simulink model "SimParking"  (R2017b)
settings: Solver=VariableStepAuto  StartTime=0.0  StopTime=1761  RelTol=1e-3
libraries: neural x1111
(part 21 of 60)

== system SimParking/10D- 100 100 100N/Layer 4/Delays 1 ==
  "p{4}" : Inport  PortDimensions=100  SampleTime=1
      mask Display: e = 0.06;c1 = [120 230 180]/255;c2 = ([120 230 180]+0)/(256+128);c3 = ([120 230 180]+128)/(256+128);patch([0 1 1 0],[0 0 1 1],c1);patch([0 1 1 1-e 1-e 0+e],[0 0 1 1-e 0+e 0+e],c2);patch([0 0 1 1-e 0+e 0+e],[0 1 1 1-e 1-e 0+e],c3);plot([0 1 1 0 0],[0 0 1 1 0]);
  mux : Mux  Inputs=1
      mask Display: e = 0.06;c1 = [120 150 230]/255;c2 = ([120 150 230]+0)/383;c3 = ([120 150 230]+128)/383;patch([0 1 1 0],[0 0 1 1],c1);patch([0 1 1 1-e 1-e 0+e],[0 0 1 1-e 0+e 0+e],c2);patch([0 0 1 1-e 0+e 0+e],[0 1 1 1-e 1-e 0+e],c3);plot([0 1 1 0 0],[0 0 1 1 0]);disp('Mux')
  "pd{4,3}" : Outport
      mask Display: e = 0.06;c1 = [120 230 180]/255;c2 = ([120 230 180]+0)/(256+128);c3 = ([120 230 180]+128)/(256+128);patch([0 1 1 0],[0 0 1 1],c1);patch([0 1 1 1-e 1-e 0+e],[0 0 1 1-e 0+e 0+e],c2);patch([0 0 1 1-e 0+e 0+e],[0 1 1 1-e 1-e 0+e],c3);plot([0 1 1 0 0],[0 0 1 1 0]);
  wires:
  "p{4}"/1 -> mux/1
  mux/1 -> "pd{4,3}"/1

== system SimParking/10D- 100 100 100N/Layer 4/LW{4,3} ==
  "ad{4,3}" : Inport  PortDimensions=100  SampleTime=1
      mask Display: e = 0.06;c1 = [120 230 180]/255;c2 = ([120 230 180]+0)/(256+128);c3 = ([120 230 180]+128)/(256+128);patch([0 1 1 0],[0 0 1 1],c1);patch([0 1 1 1-e 1-e 0+e],[0 0 1 1-e 0+e 0+e],c2);patch([0 0 1 1-e 0+e 0+e],[0 1 1 1-e 1-e 0+e],c3);plot([0 1 1 0 0],[0 0 1 1 0]);
  "IW{4,3}(1,:)'" : Constant  Value=[0.58065140864907160977992361949873156845569610595703125;-0.066112039002752365224324648806941695511341094970703125;1.0084944993814843883228604681789875030517578125;-0.9161011616738401475146247321390546858310699462890625;-0.61197886000859436084198250682675279676914215087890625;-0.96188175595466962608526273470488376915454864501953125;0.6658154478615332383384384229429997503757476806640625;0.253669306894615143033178128462168388068675994873046875;-0.047789102755492814111892840855944086797535419464111328125;0.2056930017197624582792059300118125975131988525390625;-0.788235313398349735081183098373003304004669189453125;0.81252383451202359054832413676194846630096435546875;0.880586120094551727532916629570536315441131591796875;0.310728251872029070934644323642714880406856536865234375;0.426423332746791949876552507703308947384357452392578125;-1.4378442695998241429578001771005801856517791748046875;-0.76862400698527266751369779740343801677227020263671875;-0.5367401396643509681183559223427437245845794677734375;0.1788804783596382730337381872232072055339813232421875;-0.483053438421408909420051713823340833187103271484375;0.260417950971423117767500343688880093395709991455078125;-0.63418149291668168832103447130066342651844024658203125;0.53082001579595605722516893365536816418170928955078125;0.6240704216430226214384902050369419157505035400390625;0.145969303182752307979086481282138265669345855712890625;-0.1372459925863576402083054972536046989262104034423828125;0.261788318191629232334349808297702111303806304931640625;-0.89483402758944607935376325258403085172176361083984375;0.400085557985017048476805712198256514966487884521484375;0.78620712071239751139728468842804431915283203125;-0.01616661136487627936642041959203197620809078216552734375;-0.319133591287700968397444967195042409002780914306640625;-0.5250450261200148016627053948468528687953948974609375;0.386346704245253913523328037626924924552440643310546875;-0.92227839555002699700736457089078612625598907470703125;-0.0933928000992329809815117869220557622611522674560546875;-0.0898344505816178473533994974786764942109584808349609375;0.03627984099991209132607394849401316605508327484130859375;0.213824804859598371908901981441886164247989654541015625;-0.71081554005856018019215980530134402215480804443359375;0.3213190743531277870914664163137786090373992919921875;-0.1329464050680488895750386291183531284332275390625;-0.7387626856994302659842333014239557087421417236328125;0.37941002852106742171400810548220761120319366455078125;-0.2280569383445431308476969434195780195295810699462890625;0.1898286392244080966751340611153864301741123199462890625;0.055918531953780638288353799225660623051226139068603515625;0.12618149731463901286332429663161747157573699951171875;-0.469304733579828992073856852584867738187313079833984375;0.45331359415498884146700220298953354358673095703125;-0.11241114545576184891029214441005024127662181854248046875;0.77149568550057912030837314887321554124355316162109375;0.5441020308254442827688990291790105402469635009765625;-0.4640419803997419823105019531794823706150054931640625;-0.38271541414365384259355096219223923981189727783203125;0.40045096965119475473926513586775399744510650634765625;-0.436585758458028660999872272441280074417591094970703125;0.25386907814860693033409688723622821271419525146484375;-0.56766035389141233924448215475422330200672149658203125;-0.52048171328359449372413791934377513825893402099609375;0.289118753056992250360934804120915941894054412841796875;0.52671878159851648337763663221267051994800567626953125;0.424025565251144154199636204793932847678661346435546875;0.50039389820546997800221333818626590073108673095703125;0.571703749575741770883041681372560560703277587890625;0.52096024030345289279608778088004328310489654541015625;-1.0972484302881044815336508690961636602878570556640625;0.06153350690420467117291991598904132843017578125;0.71182905044128819138649078013258986175060272216796875;0.26074983033264886866930964970379136502742767333984375 ...(+1684 chars)]
      mask Display: e = 0.06;c1 = [120 150 230]/255;c2 = ([120 150 230]+0)/383;c3 = ([120 150 230]+128)/383;patch([0 1 1 0],[0 0 1 1],c1);patch([0 1 1 1-e 1-e 0+e],[0 0 1 1-e 0+e 0+e],c2);patch([0 0 1 1-e 0+e 0+e],[0 1 1 1-e 1-e 0+e],c3);plot([0 1 1 0 0],[0 0 1 1 0]);disp('weights');
  "IW{4,3}(2,:)'" : Constant  Value=[-0.28083772557362507438227794409613125026226043701171875;0.1911231828179239811138501181630999781191349029541015625;-0.016841450868698114307075996975981979630887508392333984375;0.4554200807526946892522801135783083736896514892578125;-0.36212973128972147929260927412542514503002166748046875;0.926801320295038255636654866975732147693634033203125;-0.355877011541491594659447628146153874695301055908203125;0.85623599632160807271219482572632841765880584716796875;0.756287402546249598600525132496841251850128173828125;-0.76329298350666052730417732163914479315280914306640625;0.63733854117530286398363159605651162564754486083984375;0.4042672903227739755749325922806747257709503173828125;-0.4780073471390433592631552528473548591136932373046875;-0.131937221534901449881971302602323703467845916748046875;-0.6587661954386081486489956660079769790172576904296875;-0.29718600339096268303507031305343843996524810791015625;-0.93540001761999913565404085602494888007640838623046875;-0.08742265244954465497340123647518339566886425018310546875;-0.306646062263924379376334172775386832654476165771484375;-0.87451763711971464143601906471303664147853851318359375;-0.04505648757097936718540864831084036268293857574462890625;0.460335947203166562236020808995817787945270538330078125;0.48200862279706557789182852502563036978244781494140625;0.81126528858937041466248274446115829050540924072265625;0.2399824226288406470164460415617213584482669830322265625;-0.1364532114372762061638155728360288776457309722900390625;-0.62431239745605626723090608720667660236358642578125;-0.250277453183759102106620275662862695753574371337890625;-0.75649463044783471499243887592456303536891937255859375;-0.8071027354293196509615881950594484806060791015625;-0.81988668547972032296655697791720740497112274169921875;-0.346397032270781057849973194606718607246875762939453125;-0.69613850753986128427897028814186342060565948486328125;-0.061889165809577539878461038824752904474735260009765625;0.47120803315065062921718208599486388266086578369140625;0.664475984077461223620275632129050791263580322265625;0.76919053868027786879935092656523920595645904541015625;0.7373475303856593665585705821285955607891082763671875;-0.16740131540824532141442659849417395889759063720703125;-0.240409527967079206245415434750611893832683563232421875;-0.1888878432571026444453110570975695736706256866455078125;0.4511494636027981730563851670012809336185455322265625;-0.692506505069595323931253005866892635822296142578125;0.79259595332253141020117936932365410029888153076171875;0.05834549798658957009411807348442380316555500030517578125;0.218146587348889420265862781889154575765132904052734375;-0.43487330000348212166727535077370703220367431640625;-0.80850607656519868360334157841862179338932037353515625;-0.54179846129792108566647357292822562158107757568359375;0.497466837097404523948540600031265057623386383056640625;-0.83275723483408159442120677340426482260227203369140625;-0.313259439196460320875559091291506774723529815673828125;-0.886547609720330864746529186959378421306610107421875;-0.7377928319850972638249686497147195041179656982421875;0.638080651836896439732527142041362822055816650390625;-1.12388930157891397954017520532943308353424072265625;-0.451183937081455821438424891312024556100368499755859375;-0.36565296083570342222657245656591840088367462158203125;-0.04871739526611630621832915721824974752962589263916015625;0.037188394407745579972601746021609869785606861114501953125;0.31150569960416840675776484204106964170932769775390625;-0.400421024146174087121607954031787812709808349609375;-0.26081835772766848169368358867359347641468048095703125;-0.742413738383605359416606006561778485774993896484375;0.7547133260416567512862684452557004988193511962890625;-0.144541835839360477411474903419730253517627716064453125;0.08616651741913637641001599831724888645112514495849609375;-0.1555950992350655093243716464712633751332759857177734375;-0.707691521707175308364412558148615062236785888671875;0.241669398817072000884564886291627772152423858642578125 ...(+1713 chars)]
      mask Display: e = 0.06;c1 = [120 150 230]/255;c2 = ([120 150 230]+0)/383;c3 = ([120 150 230]+128)/383;patch([0 1 1 0],[0 0 1 1],c1);patch([0 1 1 1-e 1-e 0+e],[0 0 1 1-e 0+e 0+e],c2);patch([0 0 1 1-e 0+e 0+e],[0 1 1 1-e 1-e 0+e],c3);plot([0 1 1 0 0],[0 0 1 1 0]);disp('weights');
  "IW{4,3}(3,:)'" : Constant  Value=[0.58647591229283613234457561702583916485309600830078125;-0.421058716694428569748964719110517762601375579833984375;-0.363140636238678149450009868814959190785884857177734375;-0.59277276021908509306967971497215330600738525390625;0.2969096677158156172282588158850558102130889892578125;-0.2491574065080221223045242595617310144007205963134765625;0.37535650893653194071220013938727788627147674560546875;0.148212865982988384327967423814698122441768646240234375;-0.29856516170355840156247495542629621922969818115234375;0.9293945754498611488969572747009806334972381591796875;0.1489981292445567151450092069353559054434299468994140625;0.11265940839033698750437650915046106092631816864013671875;-0.45330747421276507136411737519665621221065521240234375;0.5760363144194726725544342116336338222026824951171875;-0.56434588292805998310797122030635364353656768798828125;0.0249158822641230674743706430263046058826148509979248046875;-0.68082550208771863697876369769801385700702667236328125;1.1419663462552616106648883942398242652416229248046875;1.7807261685693849262435151104000397026538848876953125;-0.0706122572379400403885796322356327436864376068115234375;-0.6991061021486142390557461112621240317821502685546875;-0.334253556285855124574624142042011953890323638916015625;0.3108382724079119530102843782515265047550201416015625;1.229372348117971025516226291074417531490325927734375;-0.646607456969967575588498220895417034626007080078125;0.799833159719270270215929485857486724853515625;0.016333214731824884091704319644122733734548091888427734375;-0.301023116553554459517982877514441497623920440673828125;-0.85815783800667932990080544186639599502086639404296875;-0.63198519800502872545422405892168171703815460205078125;-0.1914664333156863573748296403209678828716278076171875;-0.45487542007959780310244468637392856180667877197265625;-0.89301591847975547722171540954150259494781494140625;0.9128920064325745098443576353020034730434417724609375;-0.11745136206108615362087022049308870919048786163330078125;0.004229928866535978375373883153542919899336993694305419921875;0.6996137659099483929736607024096883833408355712890625;0.71630517481068445295733226885204203426837921142578125;0.61909419598402504192335982224904000759124755859375;-0.266136443148383416978930426921579055488109588623046875;0.41438062244503404141227065338171087205410003662109375;-0.86521500672426510103463215273222886025905609130859375;0.8140072634505541859795130221755243837833404541015625;-0.07851155592747881273307797300731181167066097259521484375;-0.1842273570680376948427436900601605884730815887451171875;0.59384671018971812994635683935484848916530609130859375;0.36193270579951597465395707331481389701366424560546875;-0.2480447945279894150782951101064099930226802825927734375;-2.059991919122229120375777711160480976104736328125;1.3488931132283827896145567137864418327808380126953125;0.01938056294047722782902809512961539439857006072998046875;0.51974751959193510320034192773164249956607818603515625;0.04771210145811023706219344830969930626451969146728515625;-0.11003832741984891085973430335798184387385845184326171875;0.497533018278228766906323699004133231937885284423828125;0.09918644012450829328120249783751205541193485260009765625;-0.4873907048366543648398874211125075817108154296875;-0.410650834199970449223116020220913924276828765869140625;-2.55308436795561188858982859528623521327972412109375;-0.330297856910869824798027138967881910502910614013671875;0.508391578700349011654679998173378407955169677734375;0.2228499914554546712519567108756746165454387664794921875;-0.0160958258229024035734777697825848008506000041961669921875;-0.2605509750811980662632549865520559251308441162109375;0.89979071375386521225436808890663087368011474609375;0.165940240490598800437993531886604614555835723876953125;0.131999678032650724635033157028374262154102325439453125;-0.10074238830830310742481259467240306548774242401123046875;0.06023401808436201765317719036829657852649688720703125;0.75028313699244442158686752009089104831218719482421875 ...(+1691 chars)]
      mask Display: e = 0.06;c1 = [120 150 230]/255;c2 = ([120 150 230]+0)/383;c3 = ([120 150 230]+128)/383;patch([0 1 1 0],[0 0 1 1],c1);patch([0 1 1 1-e 1-e 0+e],[0 0 1 1-e 0+e 0+e],c2);patch([0 0 1 1-e 0+e 0+e],[0 1 1 1-e 1-e 0+e],c3);plot([0 1 1 0 0],[0 0 1 1 0]);disp('weights');
  Mux : Mux  Inputs=3
      mask Display: e = 0.06;c1 = [120 150 230]/255;c2 = ([120 150 230]+0)/383;c3 = ([120 150 230]+128)/383;patch([0 1 1 0],[0 0 1 1],c1);patch([0 1 1 1-e 1-e 0+e],[0 0 1 1-e 0+e 0+e],c2);patch([0 0 1 1-e 0+e 0+e],[0 1 1 1-e 1-e 0+e],c3);plot([0 1 1 0 0],[0 0 1 1 0]);disp('Mux');
  dotprod1 : neural/Weight Functions/dotprod
  dotprod2 : neural/Weight Functions/dotprod
  dotprod3 : neural/Weight Functions/dotprod
  "lz{4,3}" : Outport
      mask Display: e = 0.06;c1 = [120 230 180]/255;c2 = ([120 230 180]+0)/(256+128);c3 = ([120 230 180]+128)/(256+128);patch([0 1 1 0],[0 0 1 1],c1);patch([0 1 1 1-e 1-e 0+e],[0 0 1 1-e 0+e 0+e],c2);patch([0 0 1 1-e 0+e 0+e],[0 1 1 1-e 1-e 0+e],c3);plot([0 1 1 0 0],[0 0 1 1 0]);
  wires:
  "IW{4,3}(1,:)'"/1 -> dotprod1/1
  "ad{4,3}"/1 -> dotprod1/2, dotprod2/2, dotprod3/2
  dotprod1/1 -> Mux/1
  "IW{4,3}(2,:)'"/1 -> dotprod2/1
  dotprod2/1 -> Mux/2
  "IW{4,3}(3,:)'"/1 -> dotprod3/1
  dotprod3/1 -> Mux/3
  Mux/1 -> "lz{4,3}"/1

== system SimParking/10D- 50 50 50 N/Layer 1/Delays 1 ==
  "p{1}" : Inport  PortDimensions=9  SampleTime=1
      mask Display: e = 0.06;c1 = [120 230 180]/255;c2 = ([120 230 180]+0)/(256+128);c3 = ([120 230 180]+128)/(256+128);patch([0 1 1 0],[0 0 1 1],c1);patch([0 1 1 1-e 1-e 0+e],[0 0 1 1-e 0+e 0+e],c2);patch([0 0 1 1-e 0+e 0+e],[0 1 1 1-e 1-e 0+e],c3);plot([0 1 1 0 0],[0 0 1 1 0]);
  Delay 1 : UnitDelay  InitialCondition=pi_input_1_delayed_1
      mask Display: e = 0.06;c1 = [120 150 230]/255;c2 = ([120 150 230]+0)/383;c3 = ([120 150 230]+128)/383;patch([0 1 1 0],[0 0 1 1],c1);patch([0 1 1 1-e 1-e 0+e],[0 0 1 1-e 0+e 0+e],c2);patch([0 0 1 1-e 0+e 0+e],[0 1 1 1-e 1-e 0+e],c3);plot([0 1 1 0 0],[0 0 1 1 0]);disp('D')
  Delay 10 : UnitDelay  InitialCondition=pi_input_1_delayed_10
      mask Display: e = 0.06;c1 = [120 150 230]/255;c2 = ([120 150 230]+0)/383;c3 = ([120 150 230]+128)/383;patch([0 1 1 0],[0 0 1 1],c1);patch([0 1 1 1-e 1-e 0+e],[0 0 1 1-e 0+e 0+e],c2);patch([0 0 1 1-e 0+e 0+e],[0 1 1 1-e 1-e 0+e],c3);plot([0 1 1 0 0],[0 0 1 1 0]);disp('D')
  Delay 2 : UnitDelay  InitialCondition=pi_input_1_delayed_2
      mask Display: e = 0.06;c1 = [120 150 230]/255;c2 = ([120 150 230]+0)/383;c3 = ([120 150 230]+128)/383;patch([0 1 1 0],[0 0 1 1],c1);patch([0 1 1 1-e 1-e 0+e],[0 0 1 1-e 0+e 0+e],c2);patch([0 0 1 1-e 0+e 0+e],[0 1 1 1-e 1-e 0+e],c3);plot([0 1 1 0 0],[0 0 1 1 0]);disp('D')
  Delay 3 : UnitDelay  InitialCondition=pi_input_1_delayed_3
      mask Display: e = 0.06;c1 = [120 150 230]/255;c2 = ([120 150 230]+0)/383;c3 = ([120 150 230]+128)/383;patch([0 1 1 0],[0 0 1 1],c1);patch([0 1 1 1-e 1-e 0+e],[0 0 1 1-e 0+e 0+e],c2);patch([0 0 1 1-e 0+e 0+e],[0 1 1 1-e 1-e 0+e],c3);plot([0 1 1 0 0],[0 0 1 1 0]);disp('D')
  Delay 4 : UnitDelay  InitialCondition=pi_input_1_delayed_4
      mask Display: e = 0.06;c1 = [120 150 230]/255;c2 = ([120 150 230]+0)/383;c3 = ([120 150 230]+128)/383;patch([0 1 1 0],[0 0 1 1],c1);patch([0 1 1 1-e 1-e 0+e],[0 0 1 1-e 0+e 0+e],c2);patch([0 0 1 1-e 0+e 0+e],[0 1 1 1-e 1-e 0+e],c3);plot([0 1 1 0 0],[0 0 1 1 0]);disp('D')
  Delay 5 : UnitDelay  InitialCondition=pi_input_1_delayed_5
      mask Display: e = 0.06;c1 = [120 150 230]/255;c2 = ([120 150 230]+0)/383;c3 = ([120 150 230]+128)/383;patch([0 1 1 0],[0 0 1 1],c1);patch([0 1 1 1-e 1-e 0+e],[0 0 1 1-e 0+e 0+e],c2);patch([0 0 1 1-e 0+e 0+e],[0 1 1 1-e 1-e 0+e],c3);plot([0 1 1 0 0],[0 0 1 1 0]);disp('D')
  Delay 6 : UnitDelay  InitialCondition=pi_input_1_delayed_6
      mask Display: e = 0.06;c1 = [120 150 230]/255;c2 = ([120 150 230]+0)/383;c3 = ([120 150 230]+128)/383;patch([0 1 1 0],[0 0 1 1],c1);patch([0 1 1 1-e 1-e 0+e],[0 0 1 1-e 0+e 0+e],c2);patch([0 0 1 1-e 0+e 0+e],[0 1 1 1-e 1-e 0+e],c3);plot([0 1 1 0 0],[0 0 1 1 0]);disp('D')
  Delay 7 : UnitDelay  InitialCondition=pi_input_1_delayed_7
      mask Display: e = 0.06;c1 = [120 150 230]/255;c2 = ([120 150 230]+0)/383;c3 = ([120 150 230]+128)/383;patch([0 1 1 0],[0 0 1 1],c1);patch([0 1 1 1-e 1-e 0+e],[0 0 1 1-e 0+e 0+e],c2);patch([0 0 1 1-e 0+e 0+e],[0 1 1 1-e 1-e 0+e],c3);plot([0 1 1 0 0],[0 0 1 1 0]);disp('D')
  Delay 8 : UnitDelay  InitialCondition=pi_input_1_delayed_8
      mask Display: e = 0.06;c1 = [120 150 230]/255;c2 = ([120 150 230]+0)/383;c3 = ([120 150 230]+128)/383;patch([0 1 1 0],[0 0 1 1],c1);patch([0 1 1 1-e 1-e 0+e],[0 0 1 1-e 0+e 0+e],c2);patch([0 0 1 1-e 0+e 0+e],[0 1 1 1-e 1-e 0+e],c3);plot([0 1 1 0 0],[0 0 1 1 0]);disp('D')
  Delay 9 : UnitDelay  InitialCondition=pi_input_1_delayed_9
      mask Display: e = 0.06;c1 = [120 150 230]/255;c2 = ([120 150 230]+0)/383;c3 = ([120 150 230]+128)/383;patch([0 1 1 0],[0 0 1 1],c1);patch([0 1 1 1-e 1-e 0+e],[0 0 1 1-e 0+e 0+e],c2);patch([0 0 1 1-e 0+e 0+e],[0 1 1 1-e 1-e 0+e],c3);plot([0 1 1 0 0],[0 0 1 1 0]);disp('D')
  mux : Mux  Inputs=10
      mask Display: e = 0.06;c1 = [120 150 230]/255;c2 = ([120 150 230]+0)/383;c3 = ([120 150 230]+128)/383;patch([0 1 1 0],[0 0 1 1],c1);patch([0 1 1 1-e 1-e 0+e],[0 0 1 1-e 0+e 0+e],c2);patch([0 0 1 1-e 0+e 0+e],[0 1 1 1-e 1-e 0+e],c3);plot([0 1 1 0 0],[0 0 1 1 0]);disp('Mux')
  "pd{1,1}" : Outport
      mask Display: e = 0.06;c1 = [120 230 180]/255;c2 = ([120 230 180]+0)/(256+128);c3 = ([120 230 180]+128)/(256+128);patch([0 1 1 0],[0 0 1 1],c1);patch([0 1 1 1-e 1-e 0+e],[0 0 1 1-e 0+e 0+e],c2);patch([0 0 1 1-e 0+e 0+e],[0 1 1 1-e 1-e 0+e],c3);plot([0 1 1 0 0],[0 0 1 1 0]);
  wires:
  "p{1}"/1 -> Delay 1/1
  Delay 1/1 -> Delay 2/1, mux/1
  Delay 2/1 -> Delay 3/1, mux/2
  Delay 3/1 -> Delay 4/1, mux/3
  Delay 4/1 -> Delay 5/1, mux/4
  Delay 5/1 -> Delay 6/1, mux/5
  Delay 6/1 -> Delay 7/1, mux/6
  Delay 7/1 -> Delay 8/1, mux/7
  Delay 8/1 -> Delay 9/1, mux/8
  Delay 9/1 -> Delay 10/1, mux/9
  Delay 10/1 -> mux/10
  mux/1 -> "pd{1,1}"/1
